simulink model "pet_integration_architecture"  (R2024a)
settings: Solver=FixedStepDiscrete  StartTime=0.0  StopTime=10.0  RelTol=1e-3
undefined symbols (not defined in the file or in its folder): D1, P
undefined symbols (not defined in the file): orig
(part 3 of 3)

== system pet_integration_architecture/brainstorm io/import_pet/bst_get ==
  Bus Element In1 : Inport  PortName=GlobalData
  Bus Element Out3 : Outport  PortName=DefaultFormats
  Bus Element Out2 : Outport  Port=2  PortName=LastUsedDirs
  Bus Element Out1 : Outport  Port=3  PortName=FileFilters
  Bus Element Out4 : Outport  Port=4  PortName=ProtocolInfo
  Bus Element Out5 : Outport  Port=5  PortName=ProtocolSubjects

== system pet_integration_architecture/brainstorm io/import_pet/bst_set ==
  Bus Element In3 : Inport  PortName=sPET
  Bus Element In1 : Inport  Port=2  PortName=DefaultFormats
  Bus Element In2 : Inport  Port=3  PortName=LastUsedDirs
  Bus Element Out1 : Outport  PortName=toDatabase

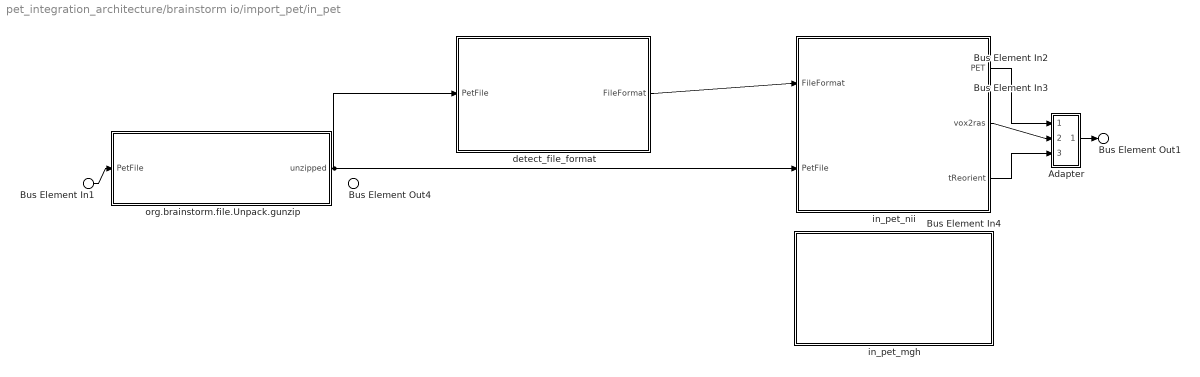
== system pet_integration_architecture/brainstorm io/import_pet/in_pet ==
  Bus Element In2 : Inport  PortName=FileFormat
  Bus Element In3 : Inport  Port=2  PortName=IsInteractive
  Bus Element In4 : Inport  Port=3  PortName=isNormalize
  Bus Element In1 : Inport  Port=4  PortName=PetFile
  Adapter : Subsystem
      settings: PortSchema="{\"entries\":[{\"content\":{\"margin\":10,\"minimumSpacing\":15,\"sides\":[{\"content\":{\"connectorIds\":[\"In1\",\"In2\",\"In3\"]},\"type\":\"ConnectorPlacement.EquallySpacedRectSide\",\"uuid\":\"b493315f-c6c8-42ab-8e4d-b8fe240af9dd\"},{\"content\":{\"connectorIds\":[\"Out1\"],\"side\":\"RIGHT\"},\"type\":\"ConnectorPlacement.EquallySpacedRectSide\",\"uuid\":\"94c0e42b-c474-4070-8a16-a26ac22942e6\"},{\"content\":{\"side\":\"TOP\"},\"type\":\"ConnectorPlacement.EquallySpacedRectSide\",\"uuid\":\"f9bc43e9-5c3a-451c-b434-9225c48927cc\"}]},\"type\":\"ConnectorPlacement.EquallySpacedConnector\",\"uuid\":\"067458af-ee7c-44e6-8802-98d558b25815\"}],\"packageUris\":[\"http://schema.mathworks.com/mf0/Connector/R2020b\"],\"version\":\"1.0\"}"
  detect_file_format : Subsystem
      settings: AttributesFormatString=%<BlockChoice>  PortSchema="{\"entries\":[{\"content\":{\"headerSize\":26,\"margin\":15,\"minimumSpacing\":25,\"sides\":[{\"content\":{\"connectorIds\":[\"In1\"]},\"type\":\"ConnectorPlacement.EquallySpacedRectSide\",\"uuid\":\"e452b68a-48a0-46a4-9e6b-6a7ab63d76ba\"},{\"content\":{\"connectorIds\":[\"Out1\"],\"side\":\"RIGHT\"},\"type\":\"ConnectorPlacement.EquallySpacedRectSide\",\"uuid\":\"bfc23a96-7562-4108-a377-c6d682106293\"},{\"content\":{\"side\":\"TOP\"},\"type\":\"ConnectorPlacement.EquallySpacedRectSide\",\"uuid\":\"898805eb-9365-4e37-9830-3cdbb7191da7\"}]},\"type\":\"ConnectorPlacement.EquallySpacedConnector\",\"uuid\":\"9a83eb3e-c81f-4df4-a7ca-e8a116b52f55\"}],\"packageUris\":[\"http://schema.mathworks.com/mf0/Connector/R2020b\"],\"version\":\"1.0\"}"
  in_pet_mgh : Subsystem  Variant=on  VariantControlMode=label  LabelModeActiveChoice=true
      settings: PortSchema="{\"entries\":[{\"content\":{\"headerSize\":38,\"margin\":15,\"minimumSpacing\":25,\"sides\":[{\"content\":{},\"type\":\"ConnectorPlacement.EquallySpacedRectSide\",\"uuid\":\"b5ae5544-e8bb-4254-ad00-58833e8a7a18\"},{\"content\":{\"side\":\"RIGHT\"},\"type\":\"ConnectorPlacement.EquallySpacedRectSide\",\"uuid\":\"fac4f2c4-a4bc-47a5-a441-dcd98ce2bd10\"},{\"content\":{\"side\":\"TOP\"},\"type\":\"ConnectorPlacement.EquallySpacedRectSide\",\"uuid\":\"59b20440-0331-47da-a238-f55a29059bc4\"}]},\"type\":\"ConnectorPlacement.EquallySpacedConnector\",\"uuid\":\"540bd42e-d22d-4480-8642-7df807d4afe7\"}],\"packageUris\":[\"http://schema.mathworks.com/mf0/Connector/R2020b\"],\"version\":\"1.0\"}"
  in_pet_nii : Subsystem
      settings: PortSchema="{\"entries\":[{\"content\":{\"headerSize\":26,\"margin\":15,\"minimumSpacing\":25,\"sides\":[{\"content\":{\"connectorIds\":[\"In1\",\"In2\"]},\"type\":\"ConnectorPlacement.EquallySpacedRectSide\",\"uuid\":\"9dc41937-0423-4f0d-95de-6a11876dea92\"},{\"content\":{\"connectorIds\":[\"Out1\",\"Out2\",\"Out3\"],\"side\":\"RIGHT\"},\"type\":\"ConnectorPlacement.EquallySpacedRectSide\",\"uuid\":\"a760f902-bb88-44c6-9e15-f93a06bbb22c\"},{\"content\":{\"side\":\"TOP\"},\"type\":\"ConnectorPlacement.EquallySpacedRectSide\",\"uuid\":\"a141426c-a194-4d5c-ba1a-f6f4f49c40a6\"}]},\"type\":\"ConnectorPlacement.EquallySpacedConnector\",\"uuid\":\"ec924d27-401c-47e0-a07a-aece678b254f\"}],\"packageUris\":[\"http://schema.mathworks.com/mf0/Connector/R2020b\"],\"version\":\"1.0\"}"
  org.brainstorm.file.Unpack.gunzip : Subsystem
      settings: PortSchema="{\"entries\":[{\"content\":{\"headerSize\":26,\"margin\":15,\"minimumSpacing\":25,\"sides\":[{\"content\":{\"connectorIds\":[\"In1\"]},\"type\":\"ConnectorPlacement.EquallySpacedRectSide\",\"uuid\":\"e452b68a-48a0-46a4-9e6b-6a7ab63d76ba\"},{\"content\":{\"connectorIds\":[\"Out1\"],\"side\":\"RIGHT\"},\"type\":\"ConnectorPlacement.EquallySpacedRectSide\",\"uuid\":\"bfc23a96-7562-4108-a377-c6d682106293\"},{\"content\":{\"side\":\"TOP\"},\"type\":\"ConnectorPlacement.EquallySpacedRectSide\",\"uuid\":\"898805eb-9365-4e37-9830-3cdbb7191da7\"},{\"content\":{\"side\":\"BOTTOM\"},\"type\":\"ConnectorPlacement.EquallySpacedRectSide\",\"uuid\":\"c4b35227-9c6e-45b4-8456-8559ba2769ae\"}]},\"type\":\"ConnectorPlacement.EquallySpacedConnector\",\"uuid\":\"9a83eb3e-c81f-4df4-a7ca-e8a116b52f55\"}],\"packageUris\":[\"http://schema.mathworks.com/mf0/Connector/R2020b\"],\"version\":\"1.0\"}"
  Bus Element Out1 : Outport  PortName=sPET
  Bus Element Out4 : Outport  Port=2  PortName=unzipped
  wires:
  Bus Element In1/1 -> org.brainstorm.file.Unpack.gunzip/1(PetFile)
  org.brainstorm.file.Unpack.gunzip/1(unzipped) -> detect_file_format/1(PetFile), in_pet_nii/2(PetFile)
  detect_file_format/1(FileFormat) -> in_pet_nii/1(FileFormat)
  in_pet_nii/1(PET) -> Adapter/1(PET)
  in_pet_nii/2(vox2ras) -> Adapter/2(vox2ras)
  in_pet_nii/3(tReorient) -> Adapter/3(tReorient)
  Adapter/1(sPET) -> Bus Element Out1/1

== system pet_integration_architecture/brainstorm io/import_pet/java_get_file ==
  Bus Element In3 : Inport  PortName=LastUsedDirs.ImportAnat
  Bus Element In1 : Inport  Port=2  PortName=PetIn
  Bus Element In4 : Inport  Port=3  PortName=Pet
  Bus Element In5 : Inport  Port=4  PortName=PET
  Bus Element In2 : Inport  Port=5  AllowServiceAccess=on  PortName=local.nifti
  Bus Element Out1 : Outport  PortName=PetFile
  Bus Element Out2 : Outport  Port=2  PortName=DefaultFormats
  Bus Element Out3 : Outport  Port=3  PortName=OutBus

== system pet_integration_architecture/brainstorm io/import_pet/out_pet_bst ==
  Bus Element In1 : Inport  PortName=sPET
  Bus Element Out1 : Outport  PortName=toFileServer

== system pet_integration_architecture/brainstorm tools/process_pet/cs_compute ==
  Bus Element In1 : Inport  PortName=PET
  Bus Element In2 : Inport  Port=2  PortName=vox2ras
  Bus Element Out1 : Outport  PortName=PetFile

== system pet_integration_architecture/brainstorm tools/process_pet/fs_align_pet ==
  Bus Element In1 : Inport  PortName=inVol
  Bus Element Out1 : Outport  PortName=fsPetFile

== system pet_integration_architecture/brainstorm tools/process_pet/fs_frame_mean ==
  Bus Element In1 : Inport  PortName=fsPetFile
  Bus Element Out1 : Outport  PortName=fsPet

== system pet_integration_architecture/brainstorm tools/process_pet/fs_register_pet ==
  Bus Element In1 : Inport  PortName=fsPetFile
  Bus Element In2 : Inport  Port=2  PortName=mri_nii
  Bus Element Out1 : Outport  PortName=fsPet

== system pet_integration_architecture/brainstorm tools/process_pet/in_pet_nii ==
  Bus Element In1 : Inport  PortName=PetFile
  Bus Element Out1 : Outport  PortName=PET
  Bus Element Out2 : Outport  Port=2  PortName=vox2ras
  Bus Element Out3 : Outport  Port=3  PortName=tReorient

== system pet_integration_architecture/brainstorm tools/process_pet/out_mri_nii ==
  Bus Element In1 : Inport  AllowServiceAccess=on  PortName=BstMriFile
  Bus Element Out1 : Outport  PortName=mri_nii

== system pet_integration_architecture/brainstorm tools/process_pet/tess_mri_mask ==
  Bus Element In1 : Inport  PortName=PetFile
  Bus Element Out1 : Outport  PortName=OutBus

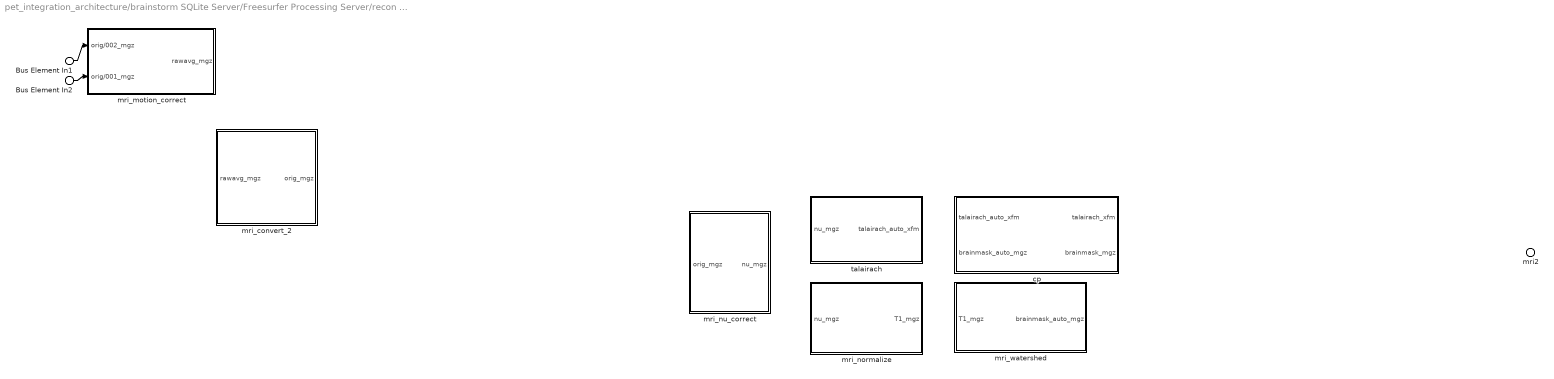
== system pet_integration_architecture/brainstorm SQLite Server/Freesurfer Processing Server/recon all/autorecon1 ==
  Bus Element In2 : Inport  PortName=orig/001_mgz
  Bus Element In1 : Inport  Port=2  PortName=orig/002_mgz
  cp : Subsystem
      settings: PortSchema="{\"entries\":[{\"content\":{\"headerSize\":26,\"margin\":15,\"minimumSpacing\":25,\"sides\":[{\"content\":{\"connectorIds\":[\"In1\",\"In2\"]},\"type\":\"ConnectorPlacement.EquallySpacedRectSide\",\"uuid\":\"d99db108-8c8a-4010-81b2-f142fbf318f5\"},{\"content\":{\"connectorIds\":[\"Out1\",\"Out2\"],\"side\":\"RIGHT\"},\"type\":\"ConnectorPlacement.EquallySpacedRectSide\",\"uuid\":\"9190d96c-22e3-4cc9-a507-8f094dc67743\"},{\"content\":{\"side\":\"TOP\"},\"type\":\"ConnectorPlacement.EquallySpacedRectSide\",\"uuid\":\"08b46875-eac1-4edb-b2eb-5598dd517a75\"}]},\"type\":\"ConnectorPlacement.EquallySpacedConnector\",\"uuid\":\"c8d2d02b-cf5a-431f-8876-22d36c8a9b33\"}],\"packageUris\":[\"http://schema.mathworks.com/mf0/Connector/R2020b\"],\"version\":\"1.0\"}"
  mri_convert_2 : Subsystem
      settings: PortSchema="{\"entries\":[{\"content\":{\"headerSize\":26,\"margin\":15,\"minimumSpacing\":25,\"sides\":[{\"content\":{\"connectorIds\":[\"In1\"]},\"type\":\"ConnectorPlacement.EquallySpacedRectSide\",\"uuid\":\"d99db108-8c8a-4010-81b2-f142fbf318f5\"},{\"content\":{\"connectorIds\":[\"Out1\"],\"side\":\"RIGHT\"},\"type\":\"ConnectorPlacement.EquallySpacedRectSide\",\"uuid\":\"9190d96c-22e3-4cc9-a507-8f094dc67743\"},{\"content\":{\"side\":\"TOP\"},\"type\":\"ConnectorPlacement.EquallySpacedRectSide\",\"uuid\":\"08b46875-eac1-4edb-b2eb-5598dd517a75\"}]},\"type\":\"ConnectorPlacement.EquallySpacedConnector\",\"uuid\":\"c8d2d02b-cf5a-431f-8876-22d36c8a9b33\"}],\"packageUris\":[\"http://schema.mathworks.com/mf0/Connector/R2020b\"],\"version\":\"1.0\"}"
  mri_motion_correct : Subsystem
      settings: PortSchema="{\"entries\":[{\"content\":{\"headerSize\":26,\"margin\":15,\"minimumSpacing\":25,\"sides\":[{\"content\":{\"connectorIds\":[\"In1\",\"In2\"]},\"type\":\"ConnectorPlacement.EquallySpacedRectSide\",\"uuid\":\"d99db108-8c8a-4010-81b2-f142fbf318f5\"},{\"content\":{\"connectorIds\":[\"Out1\"],\"side\":\"RIGHT\"},\"type\":\"ConnectorPlacement.EquallySpacedRectSide\",\"uuid\":\"9190d96c-22e3-4cc9-a507-8f094dc67743\"},{\"content\":{\"side\":\"TOP\"},\"type\":\"ConnectorPlacement.EquallySpacedRectSide\",\"uuid\":\"08b46875-eac1-4edb-b2eb-5598dd517a75\"}]},\"type\":\"ConnectorPlacement.EquallySpacedConnector\",\"uuid\":\"c8d2d02b-cf5a-431f-8876-22d36c8a9b33\"}],\"packageUris\":[\"http://schema.mathworks.com/mf0/Connector/R2020b\"],\"version\":\"1.0\"}"
  mri_normalize : Subsystem
      settings: PortSchema="{\"entries\":[{\"content\":{\"headerSize\":26,\"margin\":15,\"minimumSpacing\":25,\"sides\":[{\"content\":{\"connectorIds\":[\"In1\"]},\"type\":\"ConnectorPlacement.EquallySpacedRectSide\",\"uuid\":\"d99db108-8c8a-4010-81b2-f142fbf318f5\"},{\"content\":{\"connectorIds\":[\"Out1\"],\"side\":\"RIGHT\"},\"type\":\"ConnectorPlacement.EquallySpacedRectSide\",\"uuid\":\"9190d96c-22e3-4cc9-a507-8f094dc67743\"},{\"content\":{\"side\":\"TOP\"},\"type\":\"ConnectorPlacement.EquallySpacedRectSide\",\"uuid\":\"08b46875-eac1-4edb-b2eb-5598dd517a75\"}]},\"type\":\"ConnectorPlacement.EquallySpacedConnector\",\"uuid\":\"c8d2d02b-cf5a-431f-8876-22d36c8a9b33\"}],\"packageUris\":[\"http://schema.mathworks.com/mf0/Connector/R2020b\"],\"version\":\"1.0\"}"
  mri_nu_correct : Subsystem
      settings: PortSchema="{\"entries\":[{\"content\":{\"headerSize\":26,\"margin\":15,\"minimumSpacing\":25,\"sides\":[{\"content\":{\"connectorIds\":[\"In1\"]},\"type\":\"ConnectorPlacement.EquallySpacedRectSide\",\"uuid\":\"d99db108-8c8a-4010-81b2-f142fbf318f5\"},{\"content\":{\"connectorIds\":[\"Out1\"],\"side\":\"RIGHT\"},\"type\":\"ConnectorPlacement.EquallySpacedRectSide\",\"uuid\":\"9190d96c-22e3-4cc9-a507-8f094dc67743\"},{\"content\":{\"side\":\"TOP\"},\"type\":\"ConnectorPlacement.EquallySpacedRectSide\",\"uuid\":\"08b46875-eac1-4edb-b2eb-5598dd517a75\"}]},\"type\":\"ConnectorPlacement.EquallySpacedConnector\",\"uuid\":\"c8d2d02b-cf5a-431f-8876-22d36c8a9b33\"}],\"packageUris\":[\"http://schema.mathworks.com/mf0/Connector/R2020b\"],\"version\":\"1.0\"}"
  mri_watershed : Subsystem
      settings: PortSchema="{\"entries\":[{\"content\":{\"headerSize\":26,\"margin\":15,\"minimumSpacing\":25,\"sides\":[{\"content\":{\"connectorIds\":[\"In1\"]},\"type\":\"ConnectorPlacement.EquallySpacedRectSide\",\"uuid\":\"d99db108-8c8a-4010-81b2-f142fbf318f5\"},{\"content\":{\"connectorIds\":[\"Out1\"],\"side\":\"RIGHT\"},\"type\":\"ConnectorPlacement.EquallySpacedRectSide\",\"uuid\":\"9190d96c-22e3-4cc9-a507-8f094dc67743\"},{\"content\":{\"side\":\"TOP\"},\"type\":\"ConnectorPlacement.EquallySpacedRectSide\",\"uuid\":\"08b46875-eac1-4edb-b2eb-5598dd517a75\"}]},\"type\":\"ConnectorPlacement.EquallySpacedConnector\",\"uuid\":\"c8d2d02b-cf5a-431f-8876-22d36c8a9b33\"}],\"packageUris\":[\"http://schema.mathworks.com/mf0/Connector/R2020b\"],\"version\":\"1.0\"}"
  talairach : Subsystem
      settings: PortSchema="{\"entries\":[{\"content\":{\"headerSize\":26,\"margin\":15,\"minimumSpacing\":25,\"sides\":[{\"content\":{\"connectorIds\":[\"In1\"]},\"type\":\"ConnectorPlacement.EquallySpacedRectSide\",\"uuid\":\"d99db108-8c8a-4010-81b2-f142fbf318f5\"},{\"content\":{\"connectorIds\":[\"Out1\"],\"side\":\"RIGHT\"},\"type\":\"ConnectorPlacement.EquallySpacedRectSide\",\"uuid\":\"9190d96c-22e3-4cc9-a507-8f094dc67743\"},{\"content\":{\"side\":\"TOP\"},\"type\":\"ConnectorPlacement.EquallySpacedRectSide\",\"uuid\":\"08b46875-eac1-4edb-b2eb-5598dd517a75\"}]},\"type\":\"ConnectorPlacement.EquallySpacedConnector\",\"uuid\":\"c8d2d02b-cf5a-431f-8876-22d36c8a9b33\"}],\"packageUris\":[\"http://schema.mathworks.com/mf0/Connector/R2020b\"],\"version\":\"1.0\"}"
  mri2 : Outport  PortName=mri1
  wires:
  Bus Element In1/1 -> mri_motion_correct/1(orig/002_mgz)
  Bus Element In2/1 -> mri_motion_correct/2(orig/001_mgz)

== system pet_integration_architecture/brainstorm SQLite Server/Freesurfer Processing Server/recon all/autorecon2 ==
  Bus Element In1 : Inport  PortName=InBus

== system pet_integration_architecture/brainstorm SQLite Server/Freesurfer Processing Server/recon all/autorecon3 ==

== system pet_integration_architecture/brainstorm SQLite Server/Freesurfer Processing Server/recon all/labelDirectory ==
  Bus Element Out1 : Outport  PortName=label

== system pet_integration_architecture/brainstorm SQLite Server/Freesurfer Processing Server/recon all/mriDirectory ==
  Bus Element Out1 : Outport  PortName=mri

== system pet_integration_architecture/brainstorm SQLite Server/Freesurfer Processing Server/recon all/mri_convert ==
  Bus Element In2 : Inport  AllowServiceAccess=on  PortName=Data
  Bus Element Out2 : Outport  PortName=orig/002_mgz
  Bus Element Out1 : Outport  Port=2  PortName=orig/001_mgz

== system pet_integration_architecture/brainstorm SQLite Server/Freesurfer Processing Server/recon all/scriptsDirectory ==
  Bus Element Out1 : Outport  PortName=scripts

== system pet_integration_architecture/brainstorm SQLite Server/Freesurfer Processing Server/recon all/statsDirectory ==
  Bus Element Out1 : Outport  PortName=stats

== system pet_integration_architecture/brainstorm SQLite Server/Freesurfer Processing Server/recon all/subjectDirectory ==
  Bus Element In7 : Inport  PortName=tmp
  Bus Element In6 : Inport  Port=2  PortName=mri
  Bus Element In2 : Inport  Port=3  PortName=scripts
  Bus Element In3 : Inport  Port=4  PortName=surf
  Bus Element In1 : Inport  Port=5  PortName=stats
  Bus Element In4 : Inport  Port=6  PortName=trash
  Bus Element In5 : Inport  Port=7  PortName=label
  Bus Element Out1 : Outport  PortName=subject

== system pet_integration_architecture/brainstorm SQLite Server/Freesurfer Processing Server/recon all/surfDirectory ==
  Bus Element Out1 : Outport  PortName=surf

== system pet_integration_architecture/brainstorm SQLite Server/Freesurfer Processing Server/recon all/tmpDirectory ==
  Bus Element Out1 : Outport  PortName=tmp

== system pet_integration_architecture/brainstorm SQLite Server/Freesurfer Processing Server/recon all/trashDirectory ==
  Bus Element Out1 : Outport  PortName=trash

== system pet_integration_architecture/brainstorm database/Brainstorm metadata /Protocol/ProtocolInfo ==

== system pet_integration_architecture/brainstorm database/Brainstorm metadata /Protocol/ProtocolStudies ==

== system pet_integration_architecture/brainstorm database/Brainstorm metadata /Protocol/ProtocolSubjects ==

== system pet_integration_architecture/brainstorm io/import_pet/in_pet/Adapter ==
  In Bus Element : Inport  PortName=PET
  Bus Element In2 : Inport  Port=2  PortName=vox2ras
  Bus Element In3 : Inport  Port=3  PortName=tReorient
  Out Bus Element : Outport  PortName=sPET
  wires:
  In Bus Element/1 -> Out Bus Element/1

== system pet_integration_architecture/brainstorm io/import_pet/in_pet/detect_file_format ==
  Bus Element In1 : Inport  PortName=PetFile
  bst_fileparts : Subsystem
      settings: PortSchema="{\"entries\":[{\"content\":{\"headerSize\":26,\"margin\":15,\"minimumSpacing\":25,\"sides\":[{\"content\":{\"connectorIds\":[\"In1\"]},\"type\":\"ConnectorPlacement.EquallySpacedRectSide\",\"uuid\":\"e452b68a-48a0-46a4-9e6b-6a7ab63d76ba\"},{\"content\":{\"connectorIds\":[\"Out1\"],\"side\":\"RIGHT\"},\"type\":\"ConnectorPlacement.EquallySpacedRectSide\",\"uuid\":\"bfc23a96-7562-4108-a377-c6d682106293\"},{\"content\":{\"side\":\"TOP\"},\"type\":\"ConnectorPlacement.EquallySpacedRectSide\",\"uuid\":\"898805eb-9365-4e37-9830-3cdbb7191da7\"}]},\"type\":\"ConnectorPlacement.EquallySpacedConnector\",\"uuid\":\"9a83eb3e-c81f-4df4-a7ca-e8a116b52f55\"}],\"packageUris\":[\"http://schema.mathworks.com/mf0/Connector/R2020b\"],\"version\":\"1.0\"}"
  Bus Element Out1 : Outport  PortName=FileFormat
  wires:
  Bus Element In1/1 -> bst_fileparts/1(PetFile)
  bst_fileparts/1(fExt) -> Bus Element Out1/1

== system pet_integration_architecture/brainstorm io/import_pet/in_pet/in_pet_mgh ==
  in_pet_bst : Subsystem  VariantControl=false
      settings: PortSchema="{\"entries\":[{\"content\":{\"headerSize\":26,\"margin\":15,\"minimumSpacing\":25,\"sides\":[{\"content\":{},\"type\":\"ConnectorPlacement.EquallySpacedRectSide\",\"uuid\":\"72abe335-e3fb-41dd-b80c-12077d308238\"},{\"content\":{\"side\":\"RIGHT\"},\"type\":\"ConnectorPlacement.EquallySpacedRectSide\",\"uuid\":\"ae31e00a-5428-4492-b9cf-7f4d180b4032\"},{\"content\":{\"side\":\"TOP\"},\"type\":\"ConnectorPlacement.EquallySpacedRectSide\",\"uuid\":\"1347eab1-52cf-472f-92d5-2cceb7c753dd\"}]},\"type\":\"ConnectorPlacement.EquallySpacedConnector\",\"uuid\":\"996eae90-ea0d-4e0d-ad72-246c3f6a3cae\"}],\"packageUris\":[\"http://schema.mathworks.com/mf0/Connector/R2020b\"],\"version\":\"1.0\"}"
  in_pet_dicom : Subsystem  VariantControl=Component
      settings: PortSchema="{\"entries\":[{\"content\":{\"headerSize\":26,\"margin\":15,\"minimumSpacing\":25,\"sides\":[{\"content\":{},\"type\":\"ConnectorPlacement.EquallySpacedRectSide\",\"uuid\":\"9dc41937-0423-4f0d-95de-6a11876dea92\"},{\"content\":{\"side\":\"RIGHT\"},\"type\":\"ConnectorPlacement.EquallySpacedRectSide\",\"uuid\":\"a760f902-bb88-44c6-9e15-f93a06bbb22c\"},{\"content\":{\"side\":\"TOP\"},\"type\":\"ConnectorPlacement.EquallySpacedRectSide\",\"uuid\":\"a141426c-a194-4d5c-ba1a-f6f4f49c40a6\"}]},\"type\":\"ConnectorPlacement.EquallySpacedConnector\",\"uuid\":\"ec924d27-401c-47e0-a07a-aece678b254f\"}],\"packageUris\":[\"http://schema.mathworks.com/mf0/Connector/R2020b\"],\"version\":\"1.0\"}"
  in_pet_mgh : Subsystem  VariantControl=true
      settings: PortSchema="{\"entries\":[{\"content\":{\"headerSize\":26,\"margin\":15,\"minimumSpacing\":25,\"sides\":[{\"content\":{},\"type\":\"ConnectorPlacement.EquallySpacedRectSide\",\"uuid\":\"72abe335-e3fb-41dd-b80c-12077d308238\"},{\"content\":{\"side\":\"RIGHT\"},\"type\":\"ConnectorPlacement.EquallySpacedRectSide\",\"uuid\":\"ae31e00a-5428-4492-b9cf-7f4d180b4032\"},{\"content\":{\"side\":\"TOP\"},\"type\":\"ConnectorPlacement.EquallySpacedRectSide\",\"uuid\":\"1347eab1-52cf-472f-92d5-2cceb7c753dd\"}]},\"type\":\"ConnectorPlacement.EquallySpacedConnector\",\"uuid\":\"996eae90-ea0d-4e0d-ad72-246c3f6a3cae\"}],\"packageUris\":[\"http://schema.mathworks.com/mf0/Connector/R2020b\"],\"version\":\"1.0\"}"

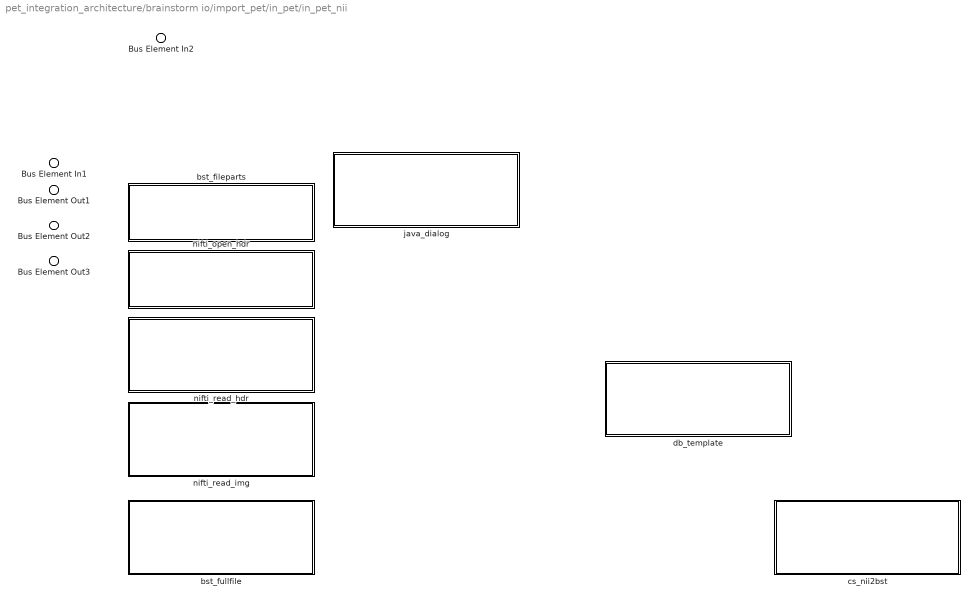
== system pet_integration_architecture/brainstorm io/import_pet/in_pet/in_pet_nii ==
  Bus Element In2 : Inport  PortName=FileFormat
  Bus Element In1 : Inport  Port=2  PortName=PetFile
  bst_fileparts : Subsystem
      settings: PortSchema="{\"entries\":[{\"content\":{\"headerSize\":26,\"margin\":15,\"minimumSpacing\":25,\"sides\":[{\"content\":{},\"type\":\"ConnectorPlacement.EquallySpacedRectSide\",\"uuid\":\"9dc41937-0423-4f0d-95de-6a11876dea92\"},{\"content\":{\"side\":\"RIGHT\"},\"type\":\"ConnectorPlacement.EquallySpacedRectSide\",\"uuid\":\"a760f902-bb88-44c6-9e15-f93a06bbb22c\"},{\"content\":{\"side\":\"TOP\"},\"type\":\"ConnectorPlacement.EquallySpacedRectSide\",\"uuid\":\"a141426c-a194-4d5c-ba1a-f6f4f49c40a6\"}]},\"type\":\"ConnectorPlacement.EquallySpacedConnector\",\"uuid\":\"ec924d27-401c-47e0-a07a-aece678b254f\"}],\"packageUris\":[\"http://schema.mathworks.com/mf0/Connector/R2020b\"],\"version\":\"1.0\"}"
  bst_fullfile : Subsystem
      settings: PortSchema="{\"entries\":[{\"content\":{\"headerSize\":26,\"margin\":15,\"minimumSpacing\":25,\"sides\":[{\"content\":{},\"type\":\"ConnectorPlacement.EquallySpacedRectSide\",\"uuid\":\"9dc41937-0423-4f0d-95de-6a11876dea92\"},{\"content\":{\"side\":\"RIGHT\"},\"type\":\"ConnectorPlacement.EquallySpacedRectSide\",\"uuid\":\"a760f902-bb88-44c6-9e15-f93a06bbb22c\"},{\"content\":{\"side\":\"TOP\"},\"type\":\"ConnectorPlacement.EquallySpacedRectSide\",\"uuid\":\"a141426c-a194-4d5c-ba1a-f6f4f49c40a6\"}]},\"type\":\"ConnectorPlacement.EquallySpacedConnector\",\"uuid\":\"ec924d27-401c-47e0-a07a-aece678b254f\"}],\"packageUris\":[\"http://schema.mathworks.com/mf0/Connector/R2020b\"],\"version\":\"1.0\"}"
  cs_nii2bst : Subsystem
      settings: PortSchema="{\"entries\":[{\"content\":{\"headerSize\":26,\"margin\":15,\"minimumSpacing\":25,\"sides\":[{\"content\":{},\"type\":\"ConnectorPlacement.EquallySpacedRectSide\",\"uuid\":\"9dc41937-0423-4f0d-95de-6a11876dea92\"},{\"content\":{\"side\":\"RIGHT\"},\"type\":\"ConnectorPlacement.EquallySpacedRectSide\",\"uuid\":\"a760f902-bb88-44c6-9e15-f93a06bbb22c\"},{\"content\":{\"side\":\"TOP\"},\"type\":\"ConnectorPlacement.EquallySpacedRectSide\",\"uuid\":\"a141426c-a194-4d5c-ba1a-f6f4f49c40a6\"}]},\"type\":\"ConnectorPlacement.EquallySpacedConnector\",\"uuid\":\"ec924d27-401c-47e0-a07a-aece678b254f\"}],\"packageUris\":[\"http://schema.mathworks.com/mf0/Connector/R2020b\"],\"version\":\"1.0\"}"
  db_template : Subsystem
      settings: PortSchema="{\"entries\":[{\"content\":{\"headerSize\":26,\"margin\":15,\"minimumSpacing\":25,\"sides\":[{\"content\":{},\"type\":\"ConnectorPlacement.EquallySpacedRectSide\",\"uuid\":\"9dc41937-0423-4f0d-95de-6a11876dea92\"},{\"content\":{\"side\":\"RIGHT\"},\"type\":\"ConnectorPlacement.EquallySpacedRectSide\",\"uuid\":\"a760f902-bb88-44c6-9e15-f93a06bbb22c\"},{\"content\":{\"side\":\"TOP\"},\"type\":\"ConnectorPlacement.EquallySpacedRectSide\",\"uuid\":\"a141426c-a194-4d5c-ba1a-f6f4f49c40a6\"}]},\"type\":\"ConnectorPlacement.EquallySpacedConnector\",\"uuid\":\"ec924d27-401c-47e0-a07a-aece678b254f\"}],\"packageUris\":[\"http://schema.mathworks.com/mf0/Connector/R2020b\"],\"version\":\"1.0\"}"
  java_dialog : Subsystem
      settings: PortSchema="{\"entries\":[{\"content\":{\"headerSize\":26,\"margin\":15,\"minimumSpacing\":25,\"sides\":[{\"content\":{},\"type\":\"ConnectorPlacement.EquallySpacedRectSide\",\"uuid\":\"9dc41937-0423-4f0d-95de-6a11876dea92\"},{\"content\":{\"side\":\"RIGHT\"},\"type\":\"ConnectorPlacement.EquallySpacedRectSide\",\"uuid\":\"a760f902-bb88-44c6-9e15-f93a06bbb22c\"},{\"content\":{\"side\":\"TOP\"},\"type\":\"ConnectorPlacement.EquallySpacedRectSide\",\"uuid\":\"a141426c-a194-4d5c-ba1a-f6f4f49c40a6\"}]},\"type\":\"ConnectorPlacement.EquallySpacedConnector\",\"uuid\":\"ec924d27-401c-47e0-a07a-aece678b254f\"}],\"packageUris\":[\"http://schema.mathworks.com/mf0/Connector/R2020b\"],\"version\":\"1.0\"}"
  nifti_open_hdr : Subsystem
      settings: PortSchema="{\"entries\":[{\"content\":{\"headerSize\":26,\"margin\":15,\"minimumSpacing\":25,\"sides\":[{\"content\":{},\"type\":\"ConnectorPlacement.EquallySpacedRectSide\",\"uuid\":\"9dc41937-0423-4f0d-95de-6a11876dea92\"},{\"content\":{\"side\":\"RIGHT\"},\"type\":\"ConnectorPlacement.EquallySpacedRectSide\",\"uuid\":\"a760f902-bb88-44c6-9e15-f93a06bbb22c\"},{\"content\":{\"side\":\"TOP\"},\"type\":\"ConnectorPlacement.EquallySpacedRectSide\",\"uuid\":\"a141426c-a194-4d5c-ba1a-f6f4f49c40a6\"}]},\"type\":\"ConnectorPlacement.EquallySpacedConnector\",\"uuid\":\"ec924d27-401c-47e0-a07a-aece678b254f\"}],\"packageUris\":[\"http://schema.mathworks.com/mf0/Connector/R2020b\"],\"version\":\"1.0\"}"
  nifti_read_hdr : Subsystem
      settings: PortSchema="{\"entries\":[{\"content\":{\"headerSize\":26,\"margin\":15,\"minimumSpacing\":25,\"sides\":[{\"content\":{},\"type\":\"ConnectorPlacement.EquallySpacedRectSide\",\"uuid\":\"9dc41937-0423-4f0d-95de-6a11876dea92\"},{\"content\":{\"side\":\"RIGHT\"},\"type\":\"ConnectorPlacement.EquallySpacedRectSide\",\"uuid\":\"a760f902-bb88-44c6-9e15-f93a06bbb22c\"},{\"content\":{\"side\":\"TOP\"},\"type\":\"ConnectorPlacement.EquallySpacedRectSide\",\"uuid\":\"a141426c-a194-4d5c-ba1a-f6f4f49c40a6\"}]},\"type\":\"ConnectorPlacement.EquallySpacedConnector\",\"uuid\":\"ec924d27-401c-47e0-a07a-aece678b254f\"}],\"packageUris\":[\"http://schema.mathworks.com/mf0/Connector/R2020b\"],\"version\":\"1.0\"}"
  nifti_read_img : Subsystem
      settings: PortSchema="{\"entries\":[{\"content\":{\"headerSize\":26,\"margin\":15,\"minimumSpacing\":25,\"sides\":[{\"content\":{},\"type\":\"ConnectorPlacement.EquallySpacedRectSide\",\"uuid\":\"9dc41937-0423-4f0d-95de-6a11876dea92\"},{\"content\":{\"side\":\"RIGHT\"},\"type\":\"ConnectorPlacement.EquallySpacedRectSide\",\"uuid\":\"a760f902-bb88-44c6-9e15-f93a06bbb22c\"},{\"content\":{\"side\":\"TOP\"},\"type\":\"ConnectorPlacement.EquallySpacedRectSide\",\"uuid\":\"a141426c-a194-4d5c-ba1a-f6f4f49c40a6\"}]},\"type\":\"ConnectorPlacement.EquallySpacedConnector\",\"uuid\":\"ec924d27-401c-47e0-a07a-aece678b254f\"}],\"packageUris\":[\"http://schema.mathworks.com/mf0/Connector/R2020b\"],\"version\":\"1.0\"}"
  Bus Element Out1 : Outport  PortName=PET
  Bus Element Out2 : Outport  Port=2  PortName=vox2ras
  Bus Element Out3 : Outport  Port=3  PortName=tReorient

== system pet_integration_architecture/brainstorm io/import_pet/in_pet/org.brainstorm.file.Unpack.gunzip ==
  Bus Element In1 : Inport  PortName=PetFile
  Bus Element Out1 : Outport  PortName=unzipped

== system pet_integration_architecture/brainstorm SQLite Server/Freesurfer Processing Server/recon all/autorecon1/cp ==
  Bus Element In1 : Inport  PortName=talairach_auto_xfm
  Bus Element In2 : Inport  Port=2  PortName=brainmask_auto_mgz
  Bus Element Out1 : Outport  PortName=talairach_xfm
  Bus Element Out2 : Outport  Port=2  PortName=brainmask_mgz

== system pet_integration_architecture/brainstorm SQLite Server/Freesurfer Processing Server/recon all/autorecon1/mri_convert_2 ==
  Bus Element In1 : Inport  PortName=rawavg_mgz
  Bus Element Out1 : Outport  PortName=orig_mgz

== system pet_integration_architecture/brainstorm SQLite Server/Freesurfer Processing Server/recon all/autorecon1/mri_motion_correct ==
  Bus Element In1 : Inport  PortName=orig/002_mgz
  Bus Element In2 : Inport  Port=2  PortName=orig/001_mgz
  Bus Element Out1 : Outport  PortName=rawavg_mgz

== system pet_integration_architecture/brainstorm SQLite Server/Freesurfer Processing Server/recon all/autorecon1/mri_normalize ==
  Bus Element In1 : Inport  PortName=nu_mgz
  Bus Element Out1 : Outport  PortName=T1_mgz

== system pet_integration_architecture/brainstorm SQLite Server/Freesurfer Processing Server/recon all/autorecon1/mri_nu_correct ==
  Bus Element In1 : Inport  PortName=orig_mgz
  Bus Element Out1 : Outport  PortName=nu_mgz

== system pet_integration_architecture/brainstorm SQLite Server/Freesurfer Processing Server/recon all/autorecon1/mri_watershed ==
  Bus Element In1 : Inport  PortName=T1_mgz
  Bus Element Out1 : Outport  PortName=brainmask_auto_mgz

== system pet_integration_architecture/brainstorm SQLite Server/Freesurfer Processing Server/recon all/autorecon1/talairach ==
  Bus Element In1 : Inport  PortName=nu_mgz
  Bus Element Out1 : Outport  PortName=talairach_auto_xfm

== system pet_integration_architecture/brainstorm io/import_pet/in_pet/detect_file_format/bst_fileparts ==
  Bus Element In1 : Inport  PortName=PetFile
  Bus Element Out1 : Outport  PortName=fExt

== system pet_integration_architecture/brainstorm io/import_pet/in_pet/in_pet_mgh/in_pet_bst ==

== system pet_integration_architecture/brainstorm io/import_pet/in_pet/in_pet_mgh/in_pet_dicom ==

== system pet_integration_architecture/brainstorm io/import_pet/in_pet/in_pet_mgh/in_pet_mgh ==

== system pet_integration_architecture/brainstorm io/import_pet/in_pet/in_pet_nii/bst_fileparts ==

== system pet_integration_architecture/brainstorm io/import_pet/in_pet/in_pet_nii/bst_fullfile ==

== system pet_integration_architecture/brainstorm io/import_pet/in_pet/in_pet_nii/cs_nii2bst ==

== system pet_integration_architecture/brainstorm io/import_pet/in_pet/in_pet_nii/db_template ==

== system pet_integration_architecture/brainstorm io/import_pet/in_pet/in_pet_nii/java_dialog ==

== system pet_integration_architecture/brainstorm io/import_pet/in_pet/in_pet_nii/nifti_open_hdr ==

== system pet_integration_architecture/brainstorm io/import_pet/in_pet/in_pet_nii/nifti_read_hdr ==

== system pet_integration_architecture/brainstorm io/import_pet/in_pet/in_pet_nii/nifti_read_img ==
